simulink model "single_cell_cordic_rotation"  (R2023a)
settings: Solver=VariableStepAuto  StartTime=0.0  StopTime=10.0  RelTol=1e-3
libraries: hdlsllib x3
settings Model: DataTypeOverride=Off  Creator=adarwish  LastModifiedBy=adarwish
settings OptimizationCC: BlockReduction=off  ConditionallyExecuteInputs=off  DefaultParameterBehavior=Inlined  InheritOutputTypeSmallerThanSingle=on
settings DebuggingCC: AlgebraicLoopMsg=none  SingleTaskRateTransMsg=error  ParameterOverflowMsg=none
settings HardwareCC: ProdBitPerPointer=32  ProdBitPerSizeT=32  ProdBitPerPtrDiffT=32  ProdLargestAtomicFloat=None  ProdIntDivRoundTo=Undefined  ProdEndianess=Unspecified  ProdWordSize=32  ProdHWDeviceType=ASIC/FPGA->ASIC/FPGA  TargetBitPerPointer=64  TargetBitPerSizeT=64  TargetBitPerPtrDiffT=64  TargetLongLongMode=on  TargetIntDivRoundTo=Zero  TargetEndianess=LittleEndian  TargetWordSize=64  TargetHWDeviceType=Custom Processor->MATLAB Host Computer  ProdEqTarget=off

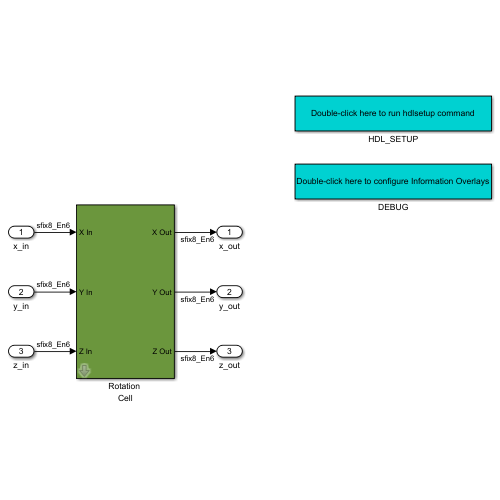
[thumbnail: Simulink's stored preview of the top-level diagram]
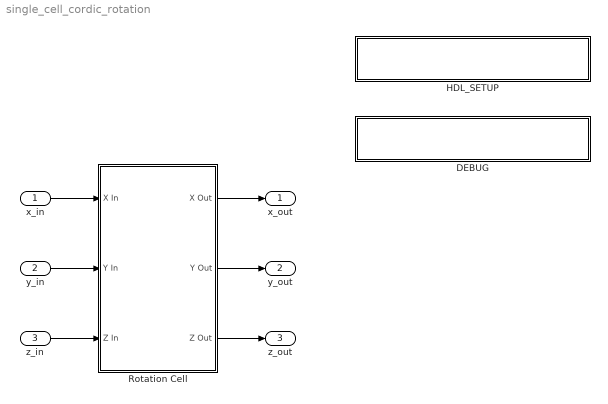
== system single_cell_cordic_rotation ==
  x_in : Inport  OutDataTypeStr=DT_X_IN  PortDimensions=1  SampleTime=[1e-08,0]
  y_in : Inport  Port=2  OutDataTypeStr=DT_Y_IN  PortDimensions=1  SampleTime=[1e-08,0]
  z_in : Inport  Port=3  OutDataTypeStr=DT_Z_IN  PortDimensions=1  SampleTime=[1e-08,0]
  DEBUG : Subsystem
      settings: OpenFcn=|
      | set_param(bdroot, 'ShowLineDimensions', 'on');
      | set_param(bdroot, 'SampleTimeColors', 'on');
      | set_param(bdroot, 'ShowLineDimensions', 'on');
      | disp('DONE Configuring Information Overlay')
      mask Display: disp(['Double-click here to configure Information Overlays'])
  HDL_SETUP : Subsystem
      settings: OpenFcn=hdlsetup(bdroot);
      mask Display: disp(['Double-click here to run hdlsetup command'])
  Rotation Cell : Subsystem  mask(Rotation Cell){i=0}
      mask prompts: i "Number of Iterations (i)"
  x_out : Outport  OutDataTypeStr=DT_X_OUT  PortDimensions=[1 1]  SampleTime=[1e-08,0]
  y_out : Outport  Port=2  OutDataTypeStr=DT_Y_OUT  PortDimensions=[1 1]  SampleTime=[1e-08,0]
  z_out : Outport  Port=3  OutDataTypeStr=DT_Z_OUT  PortDimensions=[1 1]  SampleTime=[1e-08,0]
  wires:
  x_in/1 -> Rotation Cell/1(X In)
  y_in/1 -> Rotation Cell/2(Y In)
  z_in/1 -> Rotation Cell/3(Z In)
  Rotation Cell/1(X Out) -> x_out/1
  Rotation Cell/3(Z Out) -> z_out/1
  Rotation Cell/2(Y Out) -> y_out/1

== system single_cell_cordic_rotation/DEBUG ==

== system single_cell_cordic_rotation/HDL_SETUP ==

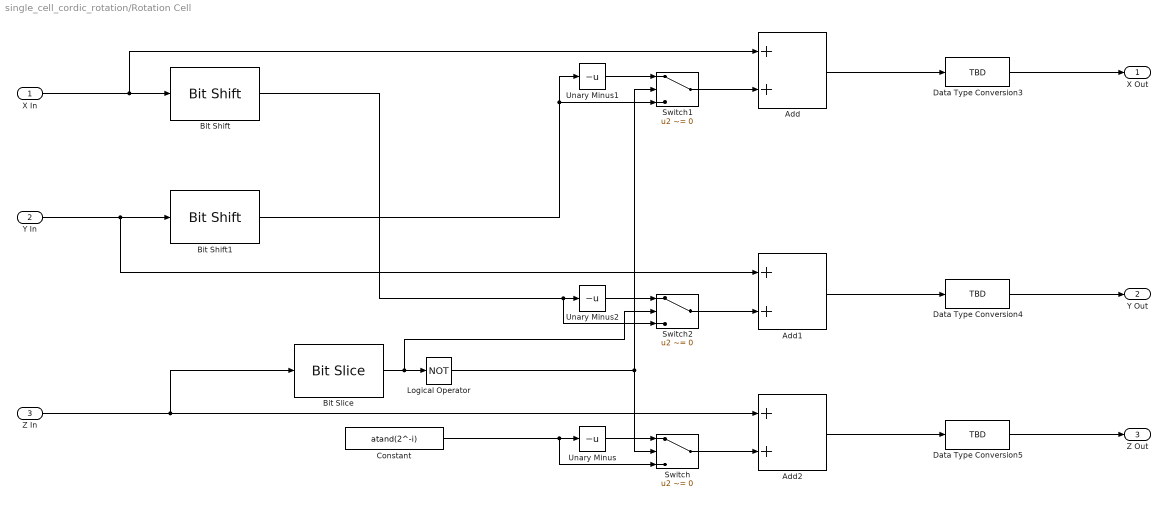
== system single_cell_cordic_rotation/Rotation Cell ==
  X In : Inport
  Y In : Inport  Port=2
  Z In : Inport  Port=3
  Add : Sum  OutDataTypeStr=Inherit: Same as first input
  Add1 : Sum  OutDataTypeStr=Inherit: Same as first input
  Add2 : Sum  OutDataTypeStr=Inherit: Same as first input
  Bit Shift : hdlsllib/Logic and Bit Operations/Bit Shift  mode=Shift Right Arithmetic  N=i
  Bit Shift1 : hdlsllib/Logic and Bit Operations/Bit Shift  mode=Shift Right Arithmetic  N=i
  Bit Slice : hdlsllib/Logic and Bit Operations/Bit Slice  lidx=TBD  ridx=TBD
  Constant : Constant  Value=atand(2^-i)  OutDataTypeStr=Inherit: Inherit via back propagation  SampleTime=-1
  Data Type Conversion3 : DataTypeConversion  OutDataTypeStr=TBD  SaturateOnIntegerOverflow=off  RndMeth=Floor
  Data Type Conversion4 : DataTypeConversion  OutDataTypeStr=TBD  SaturateOnIntegerOverflow=off  RndMeth=Floor
  Data Type Conversion5 : DataTypeConversion  OutDataTypeStr=TBD  SaturateOnIntegerOverflow=off  RndMeth=Floor
  Logical Operator : Logic  Operator=NOT  AllPortsSameDT=off  OutDataTypeStr=boolean
  Switch : Switch  Criteria=u2 ~= 0  SaturateOnIntegerOverflow=off  InputSameDT=off
  Switch1 : Switch  Criteria=u2 ~= 0  SaturateOnIntegerOverflow=off  InputSameDT=off
  Switch2 : Switch  Criteria=u2 ~= 0  SaturateOnIntegerOverflow=off  InputSameDT=off
  Unary Minus : UnaryMinus
  Unary Minus1 : UnaryMinus
  Unary Minus2 : UnaryMinus
  X Out : Outport
  Y Out : Outport  Port=2
  Z Out : Outport  Port=3
  wires:
  Constant/1 -> Unary Minus/1, Switch/3
  Y In/1 -> Bit Shift1/1, Add1/1
  X In/1 -> Bit Shift/1, Add/1
  Add/1 -> Data Type Conversion3/1
  Unary Minus2/1 -> Switch2/1
  Unary Minus/1 -> Switch/1
  Add1/1 -> Data Type Conversion4/1
  Switch1/1 -> Add/2
  Bit Shift/1 -> Switch2/3, Unary Minus2/1
  Switch2/1 -> Add1/2
  Unary Minus1/1 -> Switch1/1
  Bit Shift1/1 -> Switch1/3, Unary Minus1/1
  Z In/1 -> Bit Slice/1, Add2/1
  Bit Slice/1 -> Logical Operator/1, Switch2/2
  Switch/1 -> Add2/2
  Add2/1 -> Data Type Conversion5/1
  Logical Operator/1 -> Switch/2, Switch1/2
  Data Type Conversion3/1 -> X Out/1
  Data Type Conversion5/1 -> Z Out/1
  Data Type Conversion4/1 -> Y Out/1
